simulink model "NUDT"  (R2022b)
settings: Solver=VariableStepAuto  StartTime=0.0  StopTime=10.0  RelTol=1e-3
settings Model: Creator=gaozh  LastModifiedBy=Powehi

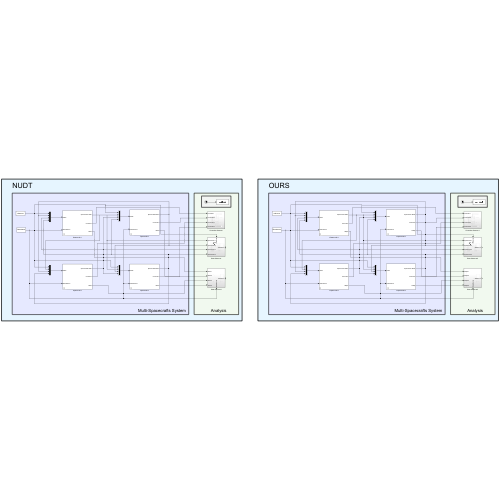
[thumbnail: Simulink's stored preview of the top-level diagram]
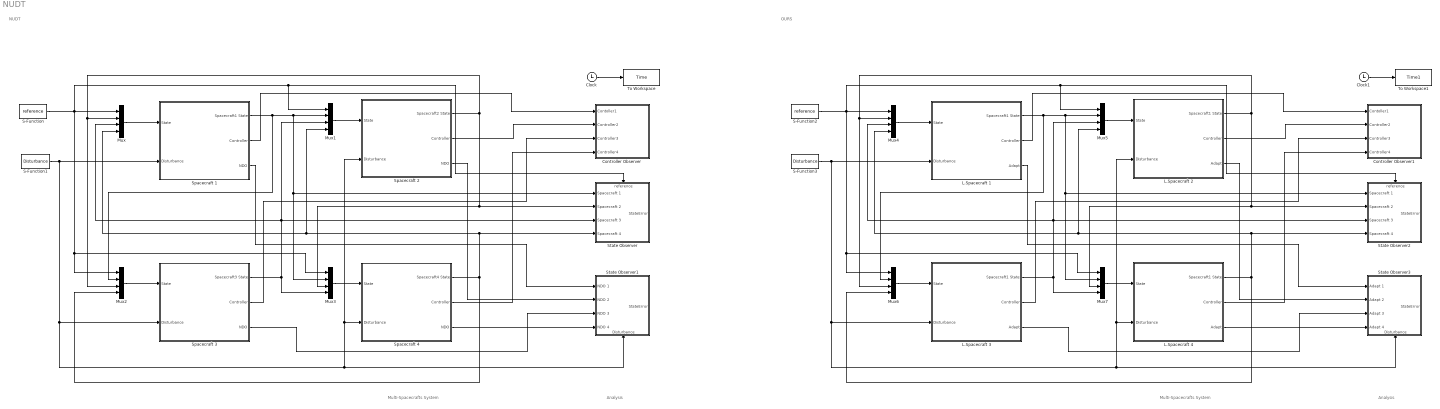
== system NUDT ==
  note: Multi-Spacecrafts System
  note: Analysis
  note: NUDT
  note: Analysis
  note: Multi-Spacecrafts System
  note: OURS
  Clock : Clock
  Clock1 : Clock
  Controller Observer : Subsystem
  Controller Observer1 : Subsystem
  L.Spacecraft 1 : Subsystem  mask{i=1, J=[0.12,0.08, 0.11, -0.05, 0.06, 0.03]}
      mask prompts: i "航天器编号"; J "航天器初始状态"
      mask DialogControl DescGroupVar Prompt: 航天器模块
      mask DialogControl DescTextVar Prompt: 其中包含航天器模型与相关控制器
      mask DialogControl ParameterGroupVar Prompt: 航天参数
  L.Spacecraft 2 : Subsystem  mask{i=2, J=[0.07,-0.13,0.12,0.04,0.05,0.02]}
      mask prompts: i "航天器编号"; J "航天器初始状态"
      mask DialogControl DescGroupVar Prompt: 航天器模块
      mask DialogControl DescTextVar Prompt: 其中包含航天器模型与相关控制器
      mask DialogControl Container3 Prompt: 航天器参数
  L.Spacecraft 3 : Subsystem  mask{i=3, J=[-0.09,0.08, 0.11, 0.06, -0.03, 0.05]}
      mask prompts: i "航天器编号"; J "航天器初始状态"
      mask DialogControl DescGroupVar Prompt: 航天器模块
      mask DialogControl DescTextVar Prompt: 其中包含航天器模型与相关控制器
      mask DialogControl ParameterGroupVar Prompt: 参数
  L.Spacecraft 4 : Subsystem  mask{i=4, J=[0.12,0.1,-0.07,0.01,0.06,-0.04]}
      mask prompts: i "航天器编号"; J "航天器初始状态"
      mask DialogControl DescGroupVar Prompt: 航天器模块
      mask DialogControl DescTextVar Prompt: 其中包含航天器模型与相关控制参数
      mask DialogControl ParameterGroupVar Prompt: 航天器参数
  Mux{,1..7} (8 alike) : Mux
  S-Function : S-Function  FunctionName=reference  SFunctionDeploymentMode=off  EnableBusSupport=off
  S-Function1 : S-Function  FunctionName=Disturbance  SFunctionDeploymentMode=off  EnableBusSupport=off
  S-Function2 : S-Function  FunctionName=reference  SFunctionDeploymentMode=off  EnableBusSupport=off
  S-Function3 : S-Function  FunctionName=Disturbance  SFunctionDeploymentMode=off  EnableBusSupport=off
  Spacecraft 1 : Subsystem  mask{i=1, J=[0.12,0.08, 0.11, -0.05, 0.06, 0.03]}
      mask prompts: i "航天器编号"; J "航天器初始状态"
      mask DialogControl DescGroupVar Prompt: 航天器模块
      mask DialogControl DescTextVar Prompt: 其中包含航天器模型与相关控制器
      mask DialogControl ParameterGroupVar Prompt: 航天参数
  Spacecraft 2 : Subsystem  mask{i=2, J=[0.07,-0.13,0.12,0.04,0.05,0.02]}
      mask prompts: i "航天器编号"; J "航天器初始状态"
      mask DialogControl DescGroupVar Prompt: 航天器模块
      mask DialogControl DescTextVar Prompt: 其中包含航天器模型与相关控制器
      mask DialogControl Container3 Prompt: 航天器参数
  Spacecraft 3 : Subsystem  mask{i=3, J=[-0.09,0.08, 0.11, 0.06, -0.03, 0.05]}
      mask prompts: i "航天器编号"; J "航天器初始状态"
      mask DialogControl DescGroupVar Prompt: 航天器模块
      mask DialogControl DescTextVar Prompt: 其中包含航天器模型与相关控制器
      mask DialogControl ParameterGroupVar Prompt: 参数
  Spacecraft 4 : Subsystem  mask{i=4, J=[0.12,0.1,-0.07,0.01,0.06,-0.04]}
      mask prompts: i "航天器编号"; J "航天器初始状态"
      mask DialogControl DescGroupVar Prompt: 航天器模块
      mask DialogControl DescTextVar Prompt: 其中包含航天器模型与相关控制参数
      mask DialogControl ParameterGroupVar Prompt: 航天器参数
  State Observer : Subsystem
      settings: PortSchema="{\"entries\":[{\"content\":{\"sides\":[{\"content\":{\"connectorIds\":[\"In1\",\"In2\",\"In3\",\"In4\"]},\"type\":\"ConnectorPlacement.EquallySpacedRectSide\",\"uuid\":\"698045ef-451e-454d-ad5b-ab39bc123777\"},{\"content\":{\"connectorIds\":[\"Out1\"],\"side\":\"RIGHT\"},\"type\":\"ConnectorPlacement.EquallySpacedRectSide\",\"uuid\":\"593868e9-aadd-4e90-afaa-605581097606\"},{\"content\":{\"connectorIds\":[\"In5\"],\"side\":\"TOP\"},\"type\":\"ConnectorPlacement.EquallySpacedRectSide\",\"uuid\":\"d3b53c66-2593-4eaf-9d4f-28486757e5e2\"}]},\"type\":\"ConnectorPlacement.EquallySpacedConnector\",\"uuid\":\"dd9f9cb3-c08e-47d5-b206-ca6443de42c5\"}],\"packageUris\":[\"http://schema.mathworks.com/mf0/Connector/R2020b\"],\"version\":\"1.0\"}"
  State Observer1 : Subsystem
      settings: PortSchema="{\"entries\":[{\"content\":{\"sides\":[{\"content\":{\"connectorIds\":[\"In1\",\"In2\",\"In3\",\"In4\"]},\"type\":\"ConnectorPlacement.EquallySpacedRectSide\",\"uuid\":\"698045ef-451e-454d-ad5b-ab39bc123777\"},{\"content\":{\"connectorIds\":[\"Out1\"],\"side\":\"RIGHT\"},\"type\":\"ConnectorPlacement.EquallySpacedRectSide\",\"uuid\":\"593868e9-aadd-4e90-afaa-605581097606\"},{\"content\":{\"connectorIds\":[],\"side\":\"TOP\"},\"type\":\"ConnectorPlacement.EquallySpacedRectSide\",\"uuid\":\"d3b53c66-2593-4eaf-9d4f-28486757e5e2\"},{\"content\":{\"connectorIds\":[\"In5\"],\"side\":\"BOTTOM\"},\"type\":\"ConnectorPlacement.EquallySpacedRectSide\",\"uuid\":\"e598e2ae-b615-49cf-ae3e-8235962c4fb0\"}]},\"type\":\"ConnectorPlacement.EquallySpacedConnector\",\"uuid\":\"dd9f9cb3-c08e-47d5-b206-ca6443de42c5\"}],\"packageUris\":[\"http://schema.mathworks.com/mf0/Connector/R2020b\"],\"version\":\"1.0\"}"
  State Observer2 : Subsystem
      settings: PortSchema="{\"entries\":[{\"content\":{\"sides\":[{\"content\":{\"connectorIds\":[\"In1\",\"In2\",\"In3\",\"In4\"]},\"type\":\"ConnectorPlacement.EquallySpacedRectSide\",\"uuid\":\"698045ef-451e-454d-ad5b-ab39bc123777\"},{\"content\":{\"connectorIds\":[\"Out1\"],\"side\":\"RIGHT\"},\"type\":\"ConnectorPlacement.EquallySpacedRectSide\",\"uuid\":\"593868e9-aadd-4e90-afaa-605581097606\"},{\"content\":{\"connectorIds\":[\"In5\"],\"side\":\"TOP\"},\"type\":\"ConnectorPlacement.EquallySpacedRectSide\",\"uuid\":\"d3b53c66-2593-4eaf-9d4f-28486757e5e2\"}]},\"type\":\"ConnectorPlacement.EquallySpacedConnector\",\"uuid\":\"dd9f9cb3-c08e-47d5-b206-ca6443de42c5\"}],\"packageUris\":[\"http://schema.mathworks.com/mf0/Connector/R2020b\"],\"version\":\"1.0\"}"
  State Observer3 : Subsystem
      settings: PortSchema="{\"entries\":[{\"content\":{\"sides\":[{\"content\":{\"connectorIds\":[\"In1\",\"In2\",\"In3\",\"In4\"]},\"type\":\"ConnectorPlacement.EquallySpacedRectSide\",\"uuid\":\"698045ef-451e-454d-ad5b-ab39bc123777\"},{\"content\":{\"connectorIds\":[\"Out1\"],\"side\":\"RIGHT\"},\"type\":\"ConnectorPlacement.EquallySpacedRectSide\",\"uuid\":\"593868e9-aadd-4e90-afaa-605581097606\"},{\"content\":{\"connectorIds\":[],\"side\":\"TOP\"},\"type\":\"ConnectorPlacement.EquallySpacedRectSide\",\"uuid\":\"d3b53c66-2593-4eaf-9d4f-28486757e5e2\"},{\"content\":{\"connectorIds\":[\"In5\"],\"side\":\"BOTTOM\"},\"type\":\"ConnectorPlacement.EquallySpacedRectSide\",\"uuid\":\"e598e2ae-b615-49cf-ae3e-8235962c4fb0\"}]},\"type\":\"ConnectorPlacement.EquallySpacedConnector\",\"uuid\":\"dd9f9cb3-c08e-47d5-b206-ca6443de42c5\"}],\"packageUris\":[\"http://schema.mathworks.com/mf0/Connector/R2020b\"],\"version\":\"1.0\"}"
  To Workspace : ToWorkspace  VariableName=Time  SampleTime=-1
  To Workspace1 : ToWorkspace  VariableName=Time1  SampleTime=-1
  wires:
  Mux/1 -> Spacecraft 1/1(State)
  Mux2/1 -> Spacecraft 3/1(State)
  Clock/1 -> To Workspace/1
  Mux1/1 -> Spacecraft 2/1(State)
  Mux3/1 -> Spacecraft 4/1(State)
  S-Function/1 -> Mux3/1, Mux2/1, State Observer/5(reference), Mux1/1, Mux/1
  Spacecraft 1/1(Spacecraft1 State) -> Mux1/2, State Observer/1(Spacecraft 1), Mux3/2, Mux2/2
  Spacecraft 2/1(Spacecraft2 State) -> Mux3/3, State Observer/2(Spacecraft 2), Mux/2, Mux2/3
  Spacecraft 3/1(Spacecraft3 State) -> Mux/3, Mux1/3, State Observer/3(Spacecraft 3), Mux3/4
  Spacecraft 4/1(Spacecraft4 State) -> Mux2/4, Mux1/4, Mux/4, State Observer/4(Spacecraft 4)
  Spacecraft 3/2(Controller) -> Controller Observer/3(Controller3)
  Spacecraft 4/2(Controller) -> Controller Observer/4(Controller4)
  Spacecraft 1/2(Controller) -> Controller Observer/1(Contoller1)
  Spacecraft 2/2(Controller) -> Controller Observer/2(Controller2)
  S-Function1/1 -> State Observer1/5(Disturbance), Spacecraft 2/2(Disturbance), Spacecraft 4/2(Disturbance), Spacecraft 3/2(Disturbance), Spacecraft 1/2(Disturbance)
  Spacecraft 1/3(NDO) -> State Observer1/1(NDO 1)
  Spacecraft 3/3(NDO) -> State Observer1/3(NDO 3)
  Spacecraft 4/3(NDO) -> State Observer1/4(NDO 4)
  Spacecraft 2/3(NDO) -> State Observer1/2(NDO 2)
  L.Spacecraft 2/3(Adapt) -> State Observer3/2(Adapt 2)
  L.Spacecraft 1/3(Adapt) -> State Observer3/1(Adapt 1)
  L.Spacecraft 3/3(Adapt) -> State Observer3/3(Adapt 3)
  Mux6/1 -> L.Spacecraft 3/1(State)
  L.Spacecraft 2/2(Controller) -> Controller Observer1/2(Controller2)
  Mux7/1 -> L.Spacecraft 4/1(State)
  L.Spacecraft 3/1(Spacecraft1 State) -> Mux4/3, Mux5/3, State Observer2/3(Spacecraft 3), Mux7/4
  L.Spacecraft 4/2(Controller) -> Controller Observer1/4(Controller4)
  L.Spacecraft 4/3(Adapt) -> State Observer3/4(Adapt 4)
  L.Spacecraft 3/2(Controller) -> Controller Observer1/3(Controller3)
  L.Spacecraft 1/2(Controller) -> Controller Observer1/1(Contoller1)
  S-Function2/1 -> Mux7/1, Mux6/1, State Observer2/5(reference), Mux5/1, Mux4/1
  Mux5/1 -> L.Spacecraft 2/1(State)
  L.Spacecraft 2/1(Spacecraft1 State) -> Mux7/3, State Observer2/2(Spacecraft 2), Mux4/2, Mux6/3
  Clock1/1 -> To Workspace1/1
  Mux4/1 -> L.Spacecraft 1/1(State)
  L.Spacecraft 4/1(Spacecraft1 State) -> Mux6/4, Mux5/4, Mux4/4, State Observer2/4(Spacecraft 4)
  S-Function3/1 -> L.Spacecraft 3/2(Disturbance), State Observer3/5(Disturbance), L.Spacecraft 4/2(Disturbance), L.Spacecraft 2/2(Disturbance), L.Spacecraft 1/2(Disturbance)
  L.Spacecraft 1/1(Spacecraft1 State) -> Mux5/2, State Observer2/1(Spacecraft 1), Mux7/2, Mux6/2

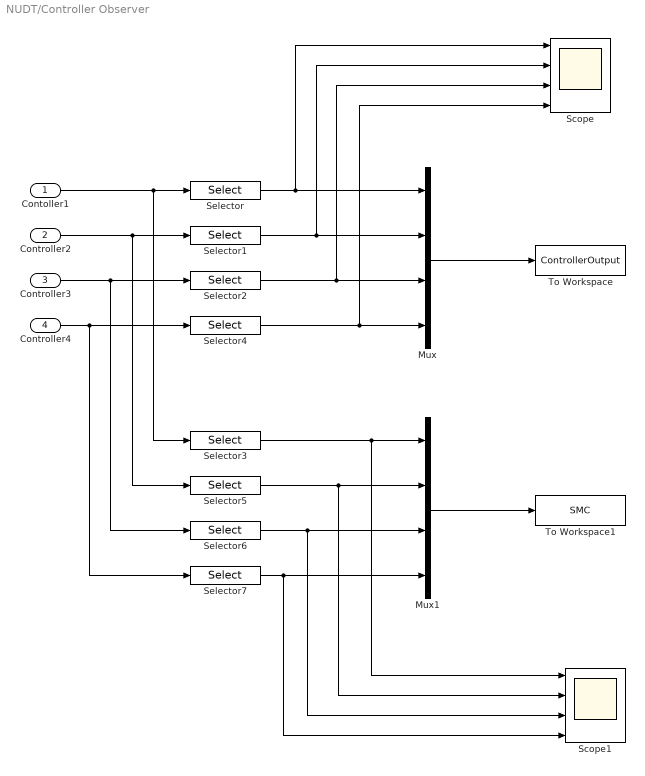
== system NUDT/Controller Observer ==
  Contoller1 : Inport
  Controller2 : Inport  Port=2
  Controller3 : Inport  Port=3
  Controller4 : Inport  Port=4
  Mux : Mux
  Mux1 : Mux
  Scope : Scope  NumInputPorts=4
  Scope1 : Scope  NumInputPorts=4
  Selector{,1..2,4} (4 alike) : Selector  InputPortWidth=6  IndexOptions=Index vector (dialog)  Indices=[1:3]  OutputSizes=1
  Selector{3,5..7} (4 alike) : Selector  InputPortWidth=6  IndexOptions=Index vector (dialog)  Indices=[4:6]  OutputSizes=1
  To Workspace : ToWorkspace  VariableName=ControllerOutput  SaveFormat=Timeseries  SampleTime=-1
  To Workspace1 : ToWorkspace  VariableName=SMC  SaveFormat=Timeseries  SampleTime=-1
  wires:
  Selector/1 -> Scope/1, Mux/1
  Contoller1/1 -> Selector3/1, Selector/1
  Controller2/1 -> Selector5/1, Selector1/1
  Selector1/1 -> Scope/2, Mux/2
  Selector2/1 -> Scope/3, Mux/3
  Controller3/1 -> Selector6/1, Selector2/1
  Controller4/1 -> Selector7/1, Selector4/1
  Selector4/1 -> Scope/4, Mux/4
  Selector7/1 -> Scope1/4, Mux1/4
  Selector3/1 -> Scope1/1, Mux1/1
  Selector5/1 -> Scope1/2, Mux1/2
  Selector6/1 -> Scope1/3, Mux1/3
  Mux/1 -> To Workspace/1
  Mux1/1 -> To Workspace1/1

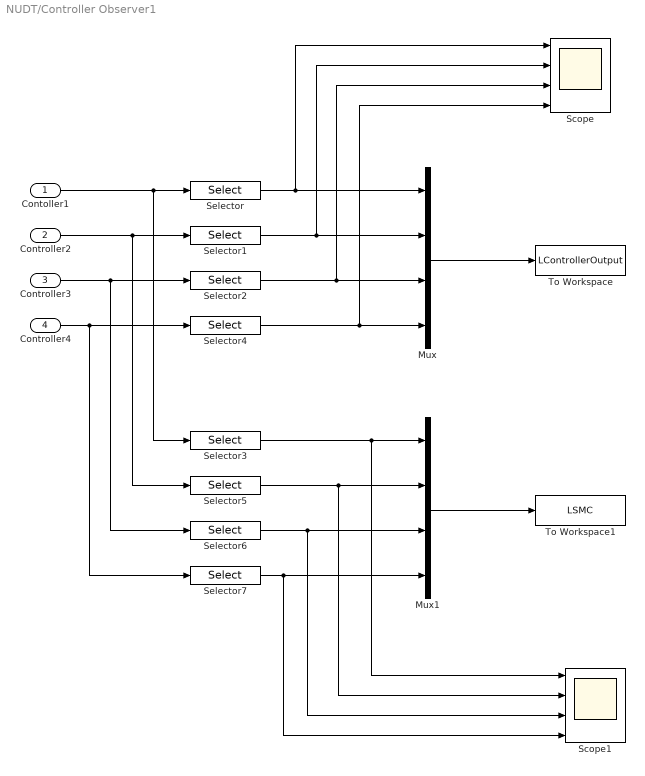
== system NUDT/Controller Observer1 ==
  Contoller1 : Inport
  Controller2 : Inport  Port=2
  Controller3 : Inport  Port=3
  Controller4 : Inport  Port=4
  Mux : Mux
  Mux1 : Mux
  Scope : Scope  NumInputPorts=4
  Scope1 : Scope  NumInputPorts=4
  Selector{,1..2,4} (4 alike) : Selector  InputPortWidth=9  IndexOptions=Index vector (dialog)  Indices=[1:3]  OutputSizes=1
  Selector{3,5..7} (4 alike) : Selector  InputPortWidth=9  IndexOptions=Index vector (dialog)  Indices=[4:9]  OutputSizes=1
  To Workspace : ToWorkspace  VariableName=LControllerOutput  SaveFormat=Timeseries  SampleTime=-1
  To Workspace1 : ToWorkspace  VariableName=LSMC  SaveFormat=Timeseries  SampleTime=-1
  wires:
  Selector/1 -> Scope/1, Mux/1
  Contoller1/1 -> Selector3/1, Selector/1
  Controller2/1 -> Selector5/1, Selector1/1
  Selector1/1 -> Scope/2, Mux/2
  Selector2/1 -> Scope/3, Mux/3
  Controller3/1 -> Selector6/1, Selector2/1
  Controller4/1 -> Selector7/1, Selector4/1
  Selector4/1 -> Scope/4, Mux/4
  Selector7/1 -> Scope1/4, Mux1/4
  Selector3/1 -> Scope1/1, Mux1/1
  Selector5/1 -> Scope1/2, Mux1/2
  Selector6/1 -> Scope1/3, Mux1/3
  Mux/1 -> To Workspace/1
  Mux1/1 -> To Workspace1/1

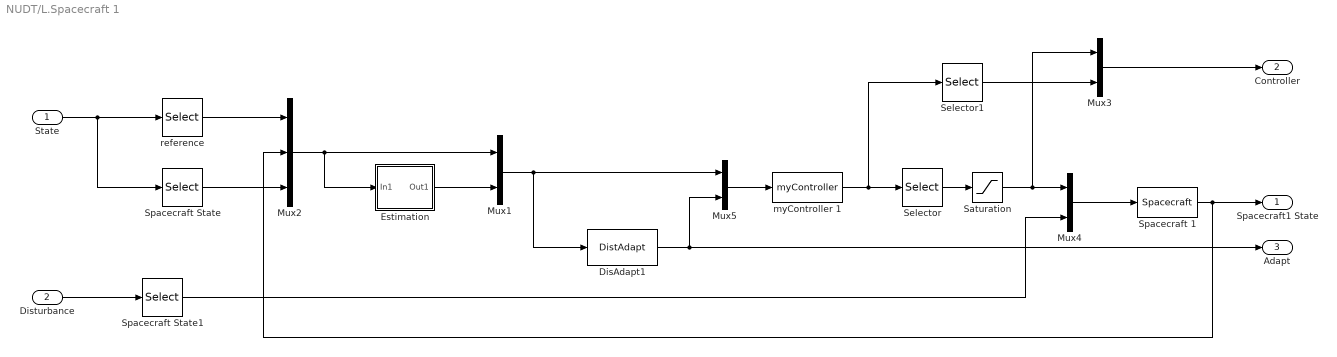
== system NUDT/L.Spacecraft 1 ==
  State : Inport
  Disturbance : Inport  Port=2
  DisAdapt1 : S-Function  FunctionName=DistAdapt  Parameters=i  SFunctionDeploymentMode=off  EnableBusSupport=off
  Estimation : Subsystem
  Mux{1,3..5} (4 alike) : Mux  Inputs=2
  Mux2 : Mux  Inputs=3
  Saturation : Saturate  UpperLimit=inf  LowerLimit=-inf
  Selector : Selector  InputPortWidth=9  IndexOptions=Index vector (dialog)  Indices=[1:3]  OutputSizes=1
  Selector1 : Selector  InputPortWidth=9  IndexOptions=Index vector (dialog)  Indices=[4:9]  OutputSizes=1
  Spacecraft 1 : S-Function  FunctionName=Spacecraft  Parameters=i,J  SFunctionDeploymentMode=off  EnableBusSupport=off
  Spacecraft State : Selector  InputPortWidth=24  IndexOptions=Index vector (dialog)  Indices=[7:24]  OutputSizes=1
  Spacecraft State1 : Selector  InputPortWidth=12  IndexOptions=Index vector (dialog)  Indices=[1:3]  OutputSizes=1
  myController 1 : S-Function  FunctionName=myController  Parameters=i  SFunctionDeploymentMode=off  EnableBusSupport=off
  reference : Selector  InputPortWidth=24  IndexOptions=Index vector (dialog)  Indices=[1:6]  OutputSizes=1
  Spacecraft1 State : Outport
  Controller : Outport  Port=2
  Adapt : Outport  Port=3
  wires:
  Selector/1 -> Saturation/1
  Mux1/1 -> Mux5/1, DisAdapt1/1
  State/1 -> Spacecraft State/1, reference/1
  reference/1 -> Mux2/1
  Spacecraft State/1 -> Mux2/3
  Saturation/1 -> Mux3/1, Mux4/1
  Mux3/1 -> Controller/1
  Selector1/1 -> Mux3/2
  Spacecraft 1/1 -> Spacecraft1 State/1, Mux2/2
  Disturbance/1 -> Spacecraft State1/1
  Mux4/1 -> Spacecraft 1/1
  Spacecraft State1/1 -> Mux4/2
  Mux2/1 -> Mux1/1, Estimation/1(In1)
  Estimation/1(Out1) -> Mux1/2
  Mux5/1 -> myController 1/1
  DisAdapt1/1 -> Adapt/1, Mux5/2
  myController 1/1 -> Selector1/1, Selector/1

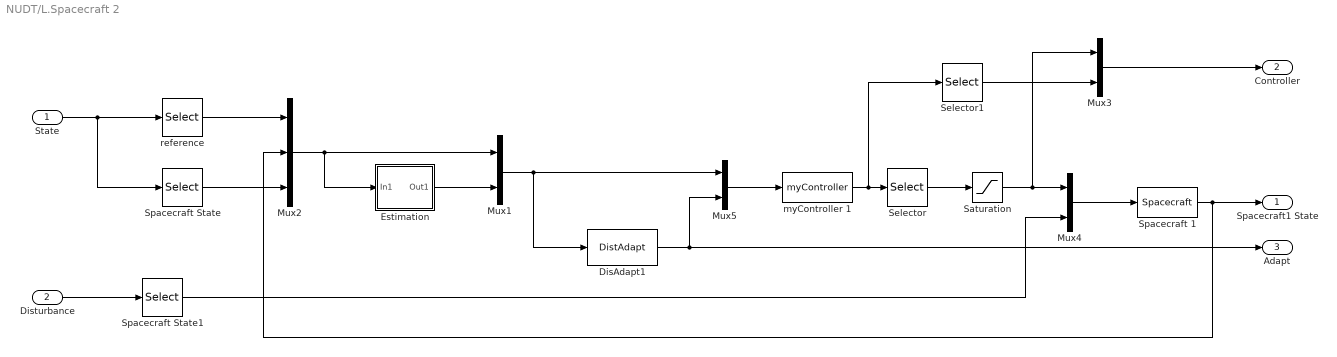
== system NUDT/L.Spacecraft 2 ==
  State : Inport
  Disturbance : Inport  Port=2
  DisAdapt1 : S-Function  FunctionName=DistAdapt  Parameters=i  SFunctionDeploymentMode=off  EnableBusSupport=off
  Estimation : Subsystem
  Mux{1,3..5} (4 alike) : Mux  Inputs=2
  Mux2 : Mux  Inputs=3
  Saturation : Saturate  UpperLimit=inf  LowerLimit=-inf
  Selector : Selector  InputPortWidth=9  IndexOptions=Index vector (dialog)  Indices=[1:3]  OutputSizes=1
  Selector1 : Selector  InputPortWidth=9  IndexOptions=Index vector (dialog)  Indices=[4:9]  OutputSizes=1
  Spacecraft 1 : S-Function  FunctionName=Spacecraft  Parameters=i,J  SFunctionDeploymentMode=off  EnableBusSupport=off
  Spacecraft State : Selector  InputPortWidth=24  IndexOptions=Index vector (dialog)  Indices=[13:24]  OutputSizes=1
  Spacecraft State1 : Selector  InputPortWidth=12  IndexOptions=Index vector (dialog)  Indices=[1:3]  OutputSizes=1
  myController 1 : S-Function  FunctionName=myController  Parameters=i  SFunctionDeploymentMode=off  EnableBusSupport=off
  reference : Selector  InputPortWidth=24  IndexOptions=Index vector (dialog)  Indices=[1:12]  OutputSizes=1
  Spacecraft1 State : Outport
  Controller : Outport  Port=2
  Adapt : Outport  Port=3
  wires:
  Mux4/1 -> Spacecraft 1/1
  myController 1/1 -> Selector1/1, Selector/1
  Selector1/1 -> Mux3/2
  Estimation/1(Out1) -> Mux1/2
  Mux1/1 -> Mux5/1, DisAdapt1/1
  Mux5/1 -> myController 1/1
  Spacecraft State1/1 -> Mux4/2
  Spacecraft 1/1 -> Spacecraft1 State/1, Mux2/2
  Disturbance/1 -> Spacecraft State1/1
  Mux3/1 -> Controller/1
  Mux2/1 -> Mux1/1, Estimation/1(In1)
  reference/1 -> Mux2/1
  Saturation/1 -> Mux3/1, Mux4/1
  Selector/1 -> Saturation/1
  DisAdapt1/1 -> Adapt/1, Mux5/2
  Spacecraft State/1 -> Mux2/3
  State/1 -> Spacecraft State/1, reference/1

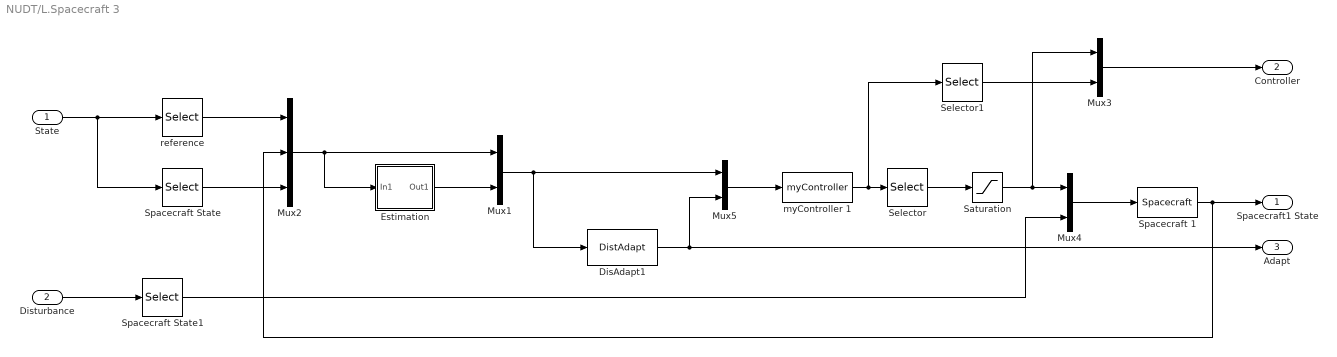
== system NUDT/L.Spacecraft 3 ==
  State : Inport
  Disturbance : Inport  Port=2
  DisAdapt1 : S-Function  FunctionName=DistAdapt  Parameters=i  SFunctionDeploymentMode=off  EnableBusSupport=off
  Estimation : Subsystem
  Mux{1,3..5} (4 alike) : Mux  Inputs=2
  Mux2 : Mux  Inputs=3
  Saturation : Saturate  UpperLimit=inf  LowerLimit=-inf
  Selector : Selector  InputPortWidth=9  IndexOptions=Index vector (dialog)  Indices=[1:3]  OutputSizes=1
  Selector1 : Selector  InputPortWidth=9  IndexOptions=Index vector (dialog)  Indices=[4:9]  OutputSizes=1
  Spacecraft 1 : S-Function  FunctionName=Spacecraft  Parameters=i,J  SFunctionDeploymentMode=off  EnableBusSupport=off
  Spacecraft State : Selector  InputPortWidth=24  IndexOptions=Index vector (dialog)  Indices=[19:24]  OutputSizes=1
  Spacecraft State1 : Selector  InputPortWidth=12  IndexOptions=Index vector (dialog)  Indices=[1:3]  OutputSizes=1
  myController 1 : S-Function  FunctionName=myController  Parameters=i  SFunctionDeploymentMode=off  EnableBusSupport=off
  reference : Selector  InputPortWidth=24  IndexOptions=Index vector (dialog)  Indices=[1:18]  OutputSizes=1
  Spacecraft1 State : Outport
  Controller : Outport  Port=2
  Adapt : Outport  Port=3
  wires:
  Mux4/1 -> Spacecraft 1/1
  myController 1/1 -> Selector1/1, Selector/1
  Selector1/1 -> Mux3/2
  Estimation/1(Out1) -> Mux1/2
  Mux1/1 -> Mux5/1, DisAdapt1/1
  Mux5/1 -> myController 1/1
  Spacecraft State1/1 -> Mux4/2
  Spacecraft 1/1 -> Spacecraft1 State/1, Mux2/2
  Disturbance/1 -> Spacecraft State1/1
  Mux3/1 -> Controller/1
  Mux2/1 -> Mux1/1, Estimation/1(In1)
  reference/1 -> Mux2/1
  Saturation/1 -> Mux3/1, Mux4/1
  Selector/1 -> Saturation/1
  DisAdapt1/1 -> Adapt/1, Mux5/2
  Spacecraft State/1 -> Mux2/3
  State/1 -> Spacecraft State/1, reference/1

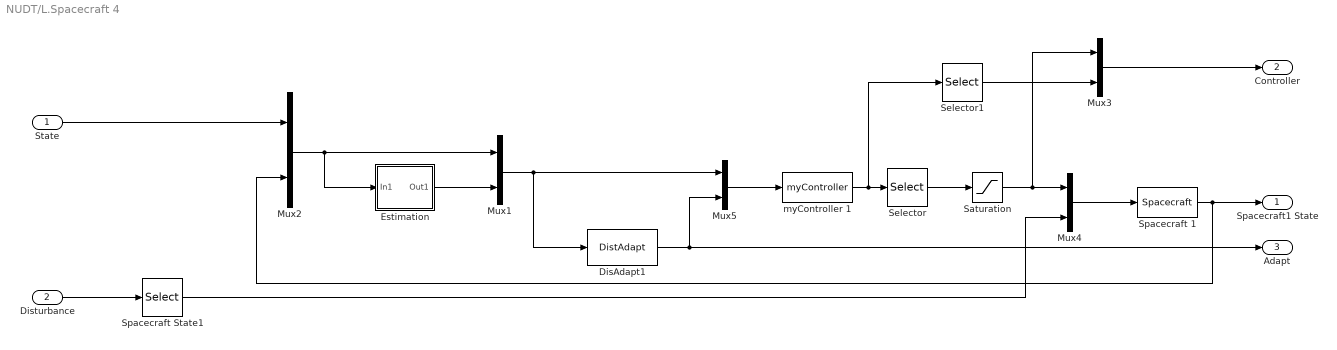
== system NUDT/L.Spacecraft 4 ==
  State : Inport
  Disturbance : Inport  Port=2
  DisAdapt1 : S-Function  FunctionName=DistAdapt  Parameters=i  SFunctionDeploymentMode=off  EnableBusSupport=off
  Estimation : Subsystem
  Mux{1..5} (5 alike) : Mux  Inputs=2
  Saturation : Saturate  UpperLimit=inf  LowerLimit=-inf
  Selector : Selector  InputPortWidth=9  IndexOptions=Index vector (dialog)  Indices=[1:3]  OutputSizes=1
  Selector1 : Selector  InputPortWidth=9  IndexOptions=Index vector (dialog)  Indices=[4:9]  OutputSizes=1
  Spacecraft 1 : S-Function  FunctionName=Spacecraft  Parameters=i,J  SFunctionDeploymentMode=off  EnableBusSupport=off
  Spacecraft State1 : Selector  InputPortWidth=12  IndexOptions=Index vector (dialog)  Indices=[1:3]  OutputSizes=1
  myController 1 : S-Function  FunctionName=myController  Parameters=i  SFunctionDeploymentMode=off  EnableBusSupport=off
  Spacecraft1 State : Outport
  Controller : Outport  Port=2
  Adapt : Outport  Port=3
  wires:
  Mux4/1 -> Spacecraft 1/1
  myController 1/1 -> Selector1/1, Selector/1
  Selector1/1 -> Mux3/2
  Estimation/1(Out1) -> Mux1/2
  Mux1/1 -> Mux5/1, DisAdapt1/1
  Mux5/1 -> myController 1/1
  Spacecraft State1/1 -> Mux4/2
  Spacecraft 1/1 -> Spacecraft1 State/1, Mux2/2
  Disturbance/1 -> Spacecraft State1/1
  Mux3/1 -> Controller/1
  Mux2/1 -> Estimation/1(In1), Mux1/1
  Saturation/1 -> Mux3/1, Mux4/1
  Selector/1 -> Saturation/1
  DisAdapt1/1 -> Adapt/1, Mux5/2
  State/1 -> Mux2/1

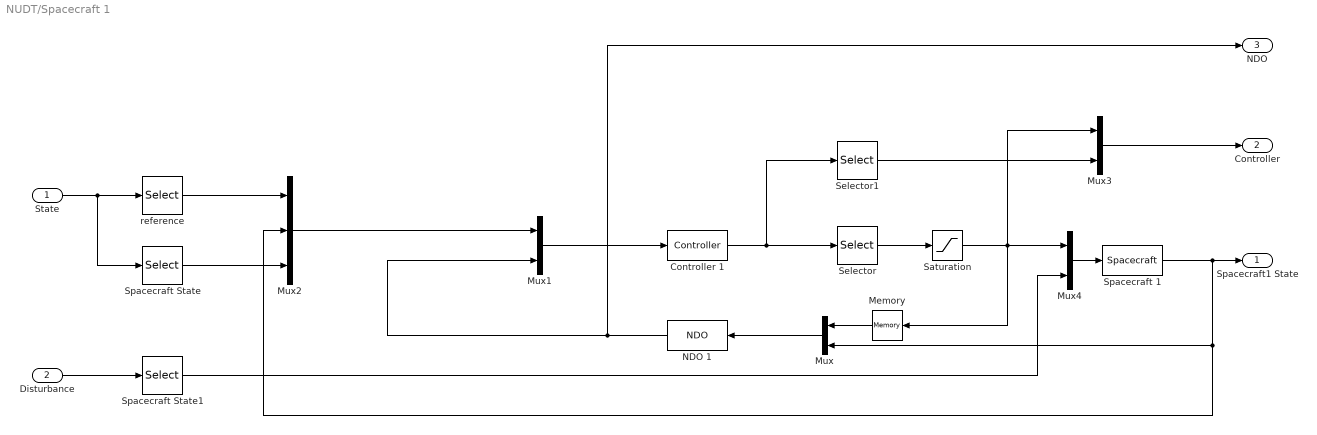
== system NUDT/Spacecraft 1 ==
  State : Inport
  Disturbance : Inport  Port=2
  Controller 1 : S-Function  FunctionName=Controller  Parameters=i  SFunctionDeploymentMode=off  EnableBusSupport=off
  Memory : Memory
  Mux{,1,3..4} (4 alike) : Mux  Inputs=2
  Mux2 : Mux  Inputs=3
  NDO 1 : S-Function  FunctionName=NDO  Parameters=i  SFunctionDeploymentMode=off  EnableBusSupport=off
  Saturation : Saturate
  Selector : Selector  InputPortWidth=6  IndexOptions=Index vector (dialog)  Indices=[1:3]  OutputSizes=1
  Selector1 : Selector  InputPortWidth=6  IndexOptions=Index vector (dialog)  Indices=[4:6]  OutputSizes=1
  Spacecraft 1 : S-Function  FunctionName=Spacecraft  Parameters=i,J  SFunctionDeploymentMode=off  EnableBusSupport=off
  Spacecraft State : Selector  InputPortWidth=24  IndexOptions=Index vector (dialog)  Indices=[7:24]  OutputSizes=1
  Spacecraft State1 : Selector  InputPortWidth=12  IndexOptions=Index vector (dialog)  Indices=[1:3]  OutputSizes=1
  reference : Selector  InputPortWidth=24  IndexOptions=Index vector (dialog)  Indices=[1:6]  OutputSizes=1
  Spacecraft1 State : Outport
  Controller : Outport  Port=2
  NDO : Outport  Port=3
  wires:
  Controller 1/1 -> Selector1/1, Selector/1
  Selector/1 -> Saturation/1
  Mux/1 -> NDO 1/1
  Mux1/1 -> Controller 1/1
  NDO 1/1 -> NDO/1, Mux1/2
  State/1 -> Spacecraft State/1, reference/1
  reference/1 -> Mux2/1
  Spacecraft State/1 -> Mux2/3
  Mux2/1 -> Mux1/1
  Saturation/1 -> Mux4/1, Memory/1, Mux3/1
  Mux3/1 -> Controller/1
  Selector1/1 -> Mux3/2
  Memory/1 -> Mux/1
  Spacecraft 1/1 -> Spacecraft1 State/1, Mux/2, Mux2/2
  Disturbance/1 -> Spacecraft State1/1
  Mux4/1 -> Spacecraft 1/1
  Spacecraft State1/1 -> Mux4/2

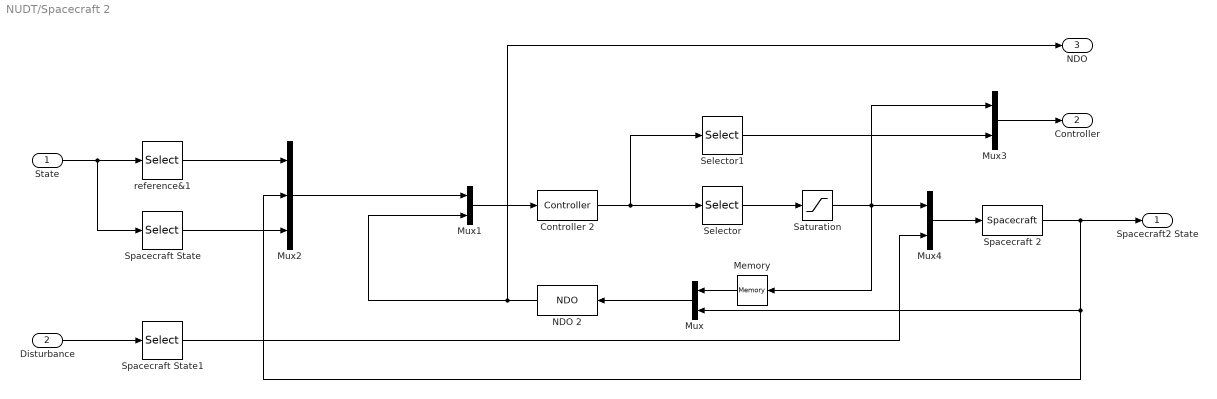
== system NUDT/Spacecraft 2 ==
  State : Inport
  Disturbance : Inport  Port=2
  Controller 2 : S-Function  FunctionName=Controller  Parameters=2  SFunctionDeploymentMode=off  EnableBusSupport=off
  Memory : Memory
  Mux{,1,3..4} (4 alike) : Mux  Inputs=2
  Mux2 : Mux  Inputs=3
  NDO 2 : S-Function  FunctionName=NDO  Parameters=2  SFunctionDeploymentMode=off  EnableBusSupport=off
  Saturation : Saturate  ZeroCross=off
  Selector : Selector  InputPortWidth=6  IndexOptions=Index vector (dialog)  Indices=[1:3]  OutputSizes=1
  Selector1 : Selector  InputPortWidth=6  IndexOptions=Index vector (dialog)  Indices=[4:6]  OutputSizes=1
  Spacecraft 2 : S-Function  FunctionName=Spacecraft  Parameters=i,J  SFunctionDeploymentMode=off  EnableBusSupport=off
  Spacecraft State : Selector  InputPortWidth=24  IndexOptions=Index vector (dialog)  Indices=[13:24]  OutputSizes=1
  Spacecraft State1 : Selector  InputPortWidth=12  IndexOptions=Index vector (dialog)  Indices=[4:6]  OutputSizes=1
  reference&1 : Selector  InputPortWidth=24  IndexOptions=Index vector (dialog)  Indices=[1:12]  OutputSizes=1
  Spacecraft2 State : Outport
  Controller : Outport  Port=2
  NDO : Outport  Port=3
  wires:
  Spacecraft 2/1 -> Mux/2, Mux2/2, Spacecraft2 State/1
  Selector/1 -> Saturation/1
  Mux/1 -> NDO 2/1
  Mux1/1 -> Controller 2/1
  State/1 -> Spacecraft State/1, reference&1/1
  Spacecraft State/1 -> Mux2/3
  reference&1/1 -> Mux2/1
  Mux2/1 -> Mux1/1
  NDO 2/1 -> NDO/1, Mux1/2
  Mux3/1 -> Controller/1
  Controller 2/1 -> Selector1/1, Selector/1
  Selector1/1 -> Mux3/2
  Memory/1 -> Mux/1
  Disturbance/1 -> Spacecraft State1/1
  Saturation/1 -> Mux4/1, Memory/1, Mux3/1
  Mux4/1 -> Spacecraft 2/1
  Spacecraft State1/1 -> Mux4/2

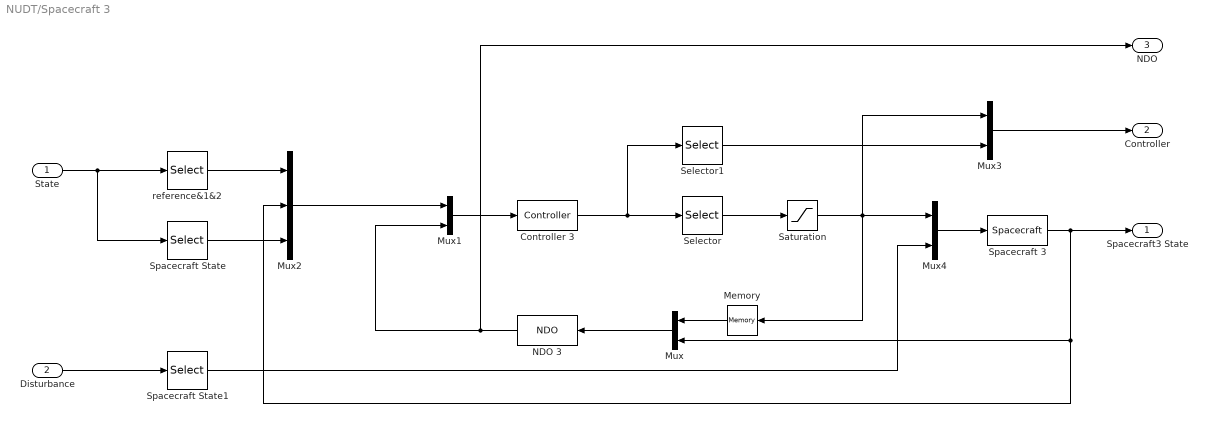
== system NUDT/Spacecraft 3 ==
  State : Inport
  Disturbance : Inport  Port=2
  Controller 3 : S-Function  FunctionName=Controller  Parameters=i  SFunctionDeploymentMode=off  EnableBusSupport=off
  Memory : Memory
  Mux{,1,3..4} (4 alike) : Mux  Inputs=2
  Mux2 : Mux  Inputs=3
  NDO 3 : S-Function  FunctionName=NDO  Parameters=i  SFunctionDeploymentMode=off  EnableBusSupport=off
  Saturation : Saturate
  Selector : Selector  InputPortWidth=6  IndexOptions=Index vector (dialog)  Indices=[1:3]  OutputSizes=1
  Selector1 : Selector  InputPortWidth=6  IndexOptions=Index vector (dialog)  Indices=[4:6]  OutputSizes=1
  Spacecraft 3 : S-Function  FunctionName=Spacecraft  Parameters=i,J  SFunctionDeploymentMode=off  EnableBusSupport=off
  Spacecraft State : Selector  InputPortWidth=24  IndexOptions=Index vector (dialog)  Indices=[19:24]  OutputSizes=1
  Spacecraft State1 : Selector  InputPortWidth=12  IndexOptions=Index vector (dialog)  Indices=[7:9]  OutputSizes=1
  reference&1&2 : Selector  InputPortWidth=24  IndexOptions=Index vector (dialog)  Indices=[1:18]  OutputSizes=1
  Spacecraft3 State : Outport
  Controller : Outport  Port=2
  NDO : Outport  Port=3
  wires:
  Spacecraft 3/1 -> Mux/2, Mux2/2, Spacecraft3 State/1
  Selector/1 -> Saturation/1
  Mux/1 -> NDO 3/1
  Mux1/1 -> Controller 3/1
  State/1 -> Spacecraft State/1, reference&1&2/1
  Spacecraft State/1 -> Mux2/3
  reference&1&2/1 -> Mux2/1
  Mux2/1 -> Mux1/1
  NDO 3/1 -> NDO/1, Mux1/2
  Selector1/1 -> Mux3/2
  Controller 3/1 -> Selector1/1, Selector/1
  Saturation/1 -> Mux4/1, Mux3/1, Memory/1
  Mux3/1 -> Controller/1
  Memory/1 -> Mux/1
  Disturbance/1 -> Spacecraft State1/1
  Mux4/1 -> Spacecraft 3/1
  Spacecraft State1/1 -> Mux4/2

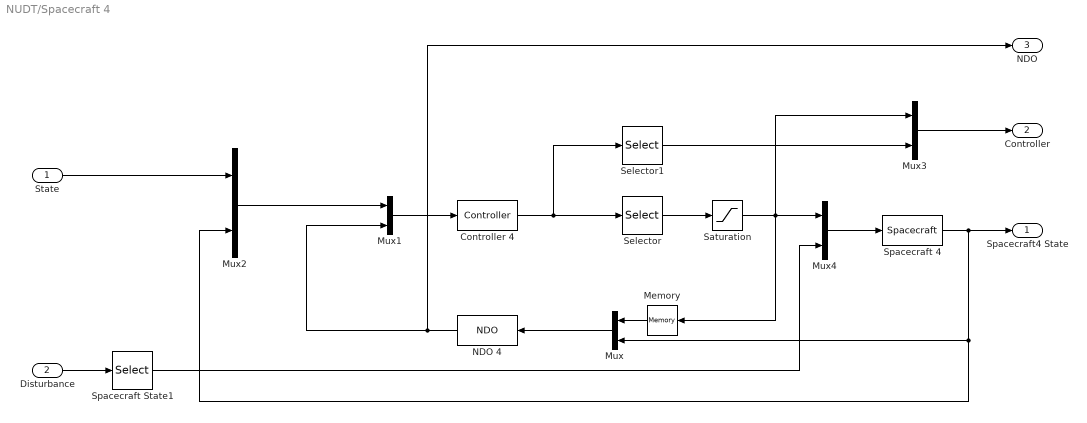
== system NUDT/Spacecraft 4 ==
  State : Inport
  Disturbance : Inport  Port=2
  Controller 4 : S-Function  FunctionName=Controller  Parameters=i  SFunctionDeploymentMode=off  EnableBusSupport=off
  Memory : Memory
  Mux{,1..4} (5 alike) : Mux  Inputs=2
  NDO 4 : S-Function  FunctionName=NDO  Parameters=i  SFunctionDeploymentMode=off  EnableBusSupport=off
  Saturation : Saturate
  Selector : Selector  InputPortWidth=6  IndexOptions=Index vector (dialog)  Indices=[1:3]  OutputSizes=1
  Selector1 : Selector  InputPortWidth=6  IndexOptions=Index vector (dialog)  Indices=[4:6]  OutputSizes=1
  Spacecraft 4 : S-Function  FunctionName=Spacecraft  Parameters=i,J  SFunctionDeploymentMode=off  EnableBusSupport=off
  Spacecraft State1 : Selector  InputPortWidth=12  IndexOptions=Index vector (dialog)  Indices=[10:12]  OutputSizes=1
  Spacecraft4 State : Outport
  Controller : Outport  Port=2
  NDO : Outport  Port=3
  wires:
  Spacecraft 4/1 -> Mux/2, Mux2/2, Spacecraft4 State/1
  Selector/1 -> Saturation/1
  Mux/1 -> NDO 4/1
  Mux1/1 -> Controller 4/1
  Mux2/1 -> Mux1/1
  NDO 4/1 -> NDO/1, Mux1/2
  State/1 -> Mux2/1
  Mux3/1 -> Controller/1
  Controller 4/1 -> Selector1/1, Selector/1
  Selector1/1 -> Mux3/2
  Saturation/1 -> Mux4/1, Memory/1, Mux3/1
  Memory/1 -> Mux/1
  Disturbance/1 -> Spacecraft State1/1
  Mux4/1 -> Spacecraft 4/1
  Spacecraft State1/1 -> Mux4/2

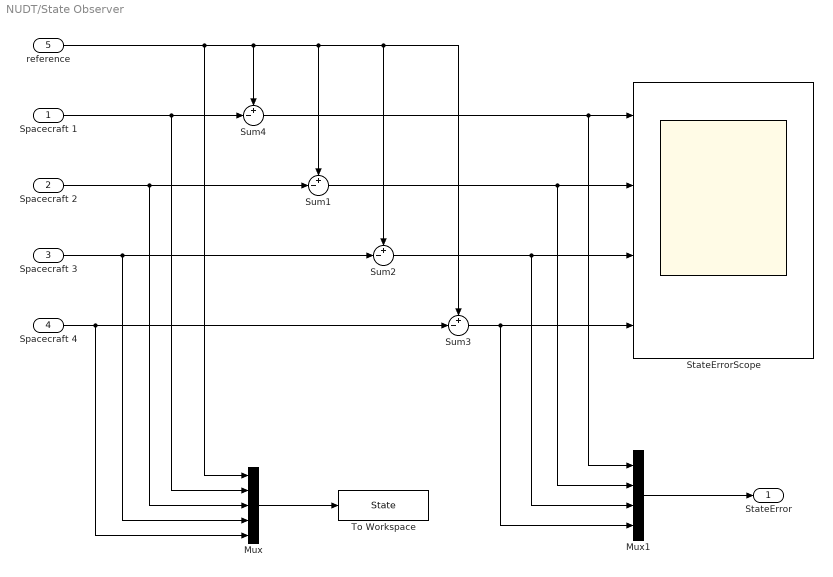
== system NUDT/State Observer ==
  Spacecraft 1 : Inport
  Spacecraft 2 : Inport  Port=2
  Spacecraft 3 : Inport  Port=3
  Spacecraft 4 : Inport  Port=4
  reference : Inport  Port=5
  Mux : Mux  Inputs=5
  Mux1 : Mux
  StateErrorScope : Scope  NumInputPorts=4
  Sum{1..4} (4 alike) : Sum  Inputs=+-|
  To Workspace : ToWorkspace  VariableName=State  SaveFormat=Timeseries  SampleTime=-1
  StateError : Outport
  wires:
  Spacecraft 1/1 -> Mux/2, Sum4/2
  Spacecraft 2/1 -> Mux/3, Sum1/2
  Spacecraft 3/1 -> Sum2/2, Mux/4
  Spacecraft 4/1 -> Mux/5, Sum3/2
  reference/1 -> Mux/1, Sum4/1, Sum1/1, Sum2/1, Sum3/1
  Mux/1 -> To Workspace/1
  Sum2/1 -> StateErrorScope/3, Mux1/3
  Sum3/1 -> StateErrorScope/4, Mux1/4
  Mux1/1 -> StateError/1
  Sum1/1 -> StateErrorScope/2, Mux1/2
  Sum4/1 -> Mux1/1, StateErrorScope/1

== system NUDT/State Observer1 ==
  NDO 1 : Inport
  NDO 2 : Inport  Port=2
  NDO 3 : Inport  Port=3
  NDO 4 : Inport  Port=4
  Disturbance : Inport  Port=5
  Mux : Mux  Inputs=5
  Mux1 : Mux
  StateErrorScope : Scope  NumInputPorts=4
  Sum{1..4} (4 alike) : Sum  Inputs=+-|
  StateError : Outport
  wires:
  Mux1/1 -> StateError/1

== system NUDT/State Observer2 ==
  Spacecraft 1 : Inport
  Spacecraft 2 : Inport  Port=2
  Spacecraft 3 : Inport  Port=3
  Spacecraft 4 : Inport  Port=4
  reference : Inport  Port=5
  Mux : Mux  Inputs=5
  Mux1 : Mux
  StateErrorScope : Scope  NumInputPorts=4
  Sum{1..4} (4 alike) : Sum  Inputs=+-|
  To Workspace : ToWorkspace  VariableName=LState  SaveFormat=Timeseries  SampleTime=-1
  StateError : Outport
  wires:
  Spacecraft 1/1 -> Mux/2, Sum4/2
  Spacecraft 2/1 -> Mux/3, Sum1/2
  Spacecraft 3/1 -> Sum2/2, Mux/4
  Spacecraft 4/1 -> Mux/5, Sum3/2
  reference/1 -> Mux/1, Sum4/1, Sum1/1, Sum2/1, Sum3/1
  Mux/1 -> To Workspace/1
  Sum2/1 -> StateErrorScope/3, Mux1/3
  Sum3/1 -> StateErrorScope/4, Mux1/4
  Mux1/1 -> StateError/1
  Sum1/1 -> StateErrorScope/2, Mux1/2
  Sum4/1 -> Mux1/1, StateErrorScope/1

== system NUDT/State Observer3 ==
  Adapt 1 : Inport
  Adapt 2 : Inport  Port=2
  Adapt 3 : Inport  Port=3
  Adapt 4 : Inport  Port=4
  Disturbance : Inport  Port=5
  Mux : Mux  Inputs=5
  Mux1 : Mux
  StateErrorScope : Scope  NumInputPorts=4
  Sum{1..4} (4 alike) : Sum  Inputs=+-|
  StateError : Outport
  wires:
  Mux1/1 -> StateError/1

== system NUDT/L.Spacecraft 1/Estimation ==
  In1 : Inport
  Derivative : Derivative  CoefficientInTFapproximation=1000
  Derivative1 : Derivative  CoefficientInTFapproximation=1000
  Mux : Mux  Inputs=2
  S-Function : S-Function  FunctionName=SFdq  Parameters=i  SFunctionDeploymentMode=off  EnableBusSupport=off
  S-Function1 : S-Function  FunctionName=SFdqd  Parameters=i  SFunctionDeploymentMode=off  EnableBusSupport=off
  Out1 : Outport
  wires:
  In1/1 -> S-Function1/1, S-Function/1
  S-Function/1 -> Derivative/1
  S-Function1/1 -> Derivative1/1
  Derivative/1 -> Mux/1
  Derivative1/1 -> Mux/2
  Mux/1 -> Out1/1

== system NUDT/L.Spacecraft 2/Estimation ==
  In1 : Inport
  Derivative : Derivative  CoefficientInTFapproximation=1000
  Derivative1 : Derivative  CoefficientInTFapproximation=1000
  Mux : Mux  Inputs=2
  S-Function : S-Function  FunctionName=SFdq  Parameters=i  SFunctionDeploymentMode=off  EnableBusSupport=off
  S-Function1 : S-Function  FunctionName=SFdqd  Parameters=i  SFunctionDeploymentMode=off  EnableBusSupport=off
  Out1 : Outport
  wires:
  In1/1 -> S-Function1/1, S-Function/1
  S-Function/1 -> Derivative/1
  S-Function1/1 -> Derivative1/1
  Derivative/1 -> Mux/1
  Derivative1/1 -> Mux/2
  Mux/1 -> Out1/1

== system NUDT/L.Spacecraft 3/Estimation ==
  In1 : Inport
  Derivative : Derivative  CoefficientInTFapproximation=1000
  Derivative1 : Derivative  CoefficientInTFapproximation=1000
  Mux : Mux  Inputs=2
  S-Function : S-Function  FunctionName=SFdq  Parameters=i  SFunctionDeploymentMode=off  EnableBusSupport=off
  S-Function1 : S-Function  FunctionName=SFdqd  Parameters=i  SFunctionDeploymentMode=off  EnableBusSupport=off
  Out1 : Outport
  wires:
  In1/1 -> S-Function1/1, S-Function/1
  S-Function/1 -> Derivative/1
  S-Function1/1 -> Derivative1/1
  Derivative/1 -> Mux/1
  Derivative1/1 -> Mux/2
  Mux/1 -> Out1/1

== system NUDT/L.Spacecraft 4/Estimation ==
  In1 : Inport
  Derivative : Derivative  CoefficientInTFapproximation=1000
  Derivative1 : Derivative  CoefficientInTFapproximation=1000
  Mux : Mux  Inputs=2
  S-Function : S-Function  FunctionName=SFdq  Parameters=i  SFunctionDeploymentMode=off  EnableBusSupport=off
  S-Function1 : S-Function  FunctionName=SFdqd  Parameters=i  SFunctionDeploymentMode=off  EnableBusSupport=off
  Out1 : Outport
  wires:
  In1/1 -> S-Function1/1, S-Function/1
  S-Function/1 -> Derivative/1
  S-Function1/1 -> Derivative1/1
  Derivative/1 -> Mux/1
  Derivative1/1 -> Mux/2
  Mux/1 -> Out1/1
